simulink library "dfr"  (Simulink 8.2)
settings: Solver=ode45  SolverMode=SingleTasking  StartTime=0.0  StopTime=10.0  RelTol=1e-3
undefined symbols (not defined in the file or in its folder): ENUM_FCWSTATE_HAPTIC_ON, FALSE, KJUD_ACCMaxTimeGap_s, KJUD_ACCMediumTimeGap_s, KJUD_ACCMinTimeGap_s, KJUD_ACCShortTimeGap_s
libraries: simulink x3
settings Model: Creator=13192  LastModifiedBy=14069

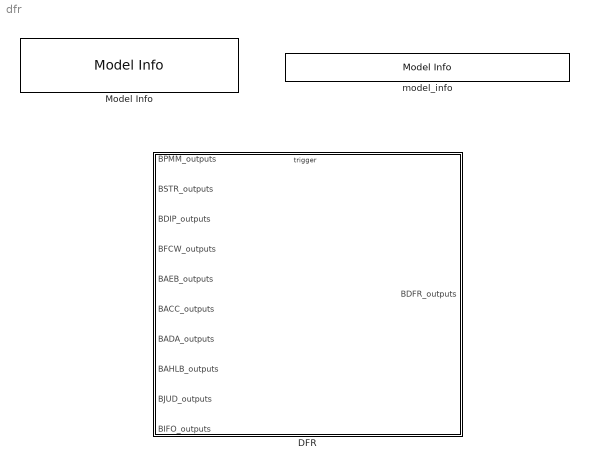
== system dfr ==
  DFR : Subsystem
      settings: RTWSystemCode=Nonreusable function  RTWFcnNameOpts=Use subsystem name  RTWFileNameOpts=Use subsystem name
  Model Info : simulink/Model-Wide Utilities/Model Info  InitialBlockCM=None  BlockCM=None  Frame=on  DisplayStringWithTags=|  HorizontalTextAlignment=Left  LeftAlignmentValue=0.02  SourceBlockDiagram=dfr  TagMaxNumber=20
      | Model Version        : %<ModelVersion>
      | Creator                   : %<Creator>
      | Last Modified by    : %<LastModifiedBy>
  model_info : simulink/Model-Wide Utilities/Model Info  InitialBlockCM=None  BlockCM=None  Frame=on  DisplayStringWithTags=$Id: hcu_lib.mdl 289 2016-04-11 06:01:08Z chimotsai $  HorizontalTextAlignment=Center  LeftAlignmentValue=0.5  SourceBlockDiagram=dfr  TagMaxNumber=20

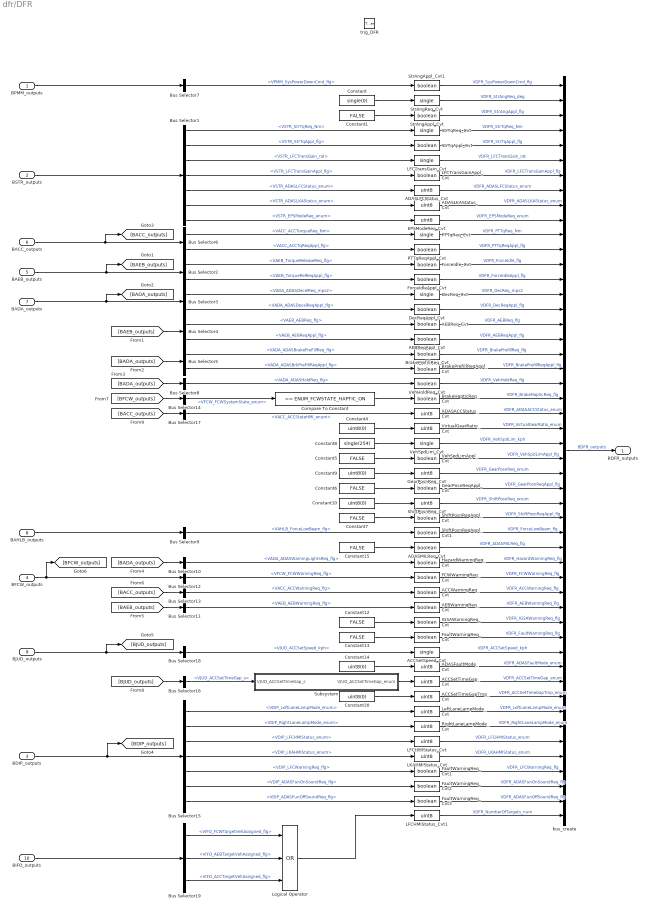
== system dfr/DFR ==
  BPMM_outputs : Inport  OutDataTypeStr=Bus: BPMM_outputs
  BSTR_outputs : Inport  Port=2  OutDataTypeStr=Bus: BSTR_outputs
  BDIP_outputs : Inport  Port=3  OutDataTypeStr=Bus: BDIP_outputs
  BFCW_outputs : Inport  Port=4  OutDataTypeStr=Bus: BFCW_outputs
  BAEB_outputs : Inport  Port=5  OutDataTypeStr=Bus: BAEB_outputs
  BACC_outputs : Inport  Port=6  OutDataTypeStr=Bus: BACC_outputs
  BADA_outputs : Inport  Port=7  OutDataTypeStr=Bus: BADA_outputs
  BAHLB_outputs : Inport  Port=8  OutDataTypeStr=Bus: BAHLB_outputs
  BJUD_outputs : Inport  Port=9  OutDataTypeStr=Bus: BJUD_outputs
  BIFO_outputs : Inport  Port=10  OutDataTypeStr=Bus: BIFO_outputs
  trig_DFR : TriggerPort  TriggerType=function-call
  ACCSetSpeed_Cvt : DataTypeConversion  OutDataTypeStr=single  SaturateOnIntegerOverflow=on  RndMeth=Zero
  ACCSetTimeGapTmp_Cvt : DataTypeConversion  OutDataTypeStr=uint8  SaturateOnIntegerOverflow=on  RndMeth=Zero
  ACCSetTimeGap_Cvt : DataTypeConversion  OutDataTypeStr=uint8  SaturateOnIntegerOverflow=on  RndMeth=Zero
  ACCWarningReq_Cvt : DataTypeConversion  OutDataTypeStr=boolean  SaturateOnIntegerOverflow=on  RndMeth=Zero
  ADASACCStatus_Cvt : DataTypeConversion  OutDataTypeStr=uint8  SaturateOnIntegerOverflow=on  RndMeth=Zero
  ADASFaultMode_Cvt : DataTypeConversion  OutDataTypeStr=uint8  SaturateOnIntegerOverflow=on  RndMeth=Zero
  ADASLFCStatus_Cvt : DataTypeConversion  OutDataTypeStr=uint8  SaturateOnIntegerOverflow=on  RndMeth=Zero
  ADASLKAStatus_Cvt : DataTypeConversion  OutDataTypeStr=uint8  SaturateOnIntegerOverflow=on  RndMeth=Zero
  ADASMILReq_Cvt : DataTypeConversion  OutDataTypeStr=boolean  SaturateOnIntegerOverflow=on  RndMeth=Zero
  AEBReqAppl_Cvt : DataTypeConversion  OutDataTypeStr=boolean  SaturateOnIntegerOverflow=on  RndMeth=Zero
  AEBReq_Cvt : DataTypeConversion  OutDataTypeStr=boolean  SaturateOnIntegerOverflow=on  RndMeth=Zero
  AEBWarningReq_Cvt : DataTypeConversion  OutDataTypeStr=boolean  SaturateOnIntegerOverflow=on  RndMeth=Zero
  BrakeHapticReq_Cvt : DataTypeConversion  OutDataTypeStr=boolean  SaturateOnIntegerOverflow=on  RndMeth=Zero
  BrakePrefillReqAppl_Cvt : DataTypeConversion  OutDataTypeStr=boolean  SaturateOnIntegerOverflow=on  RndMeth=Zero
  BrakePrefillReq_Cvt : DataTypeConversion  OutDataTypeStr=boolean  SaturateOnIntegerOverflow=on  RndMeth=Zero
  Bus Selector1 : BusSelector  OutputSignals=VSTR_StrTqReq_Nm,VSTR_StrTqAppl_flg,VSTR_LFCTransGain_rat,VSTR_LFCTransGainAppl_flg,VSTR_ADASLFCStatus_enum,VSTR_ADASLKAStatus_enum,VSTR_EPSModeReq_enum
  Bus Selector10 : BusSelector  OutputSignals=VADA_ADASWarningLightsReq_flg
  Bus Selector11 : BusSelector  OutputSignals=VAEB_AEBWarningReq_flg
  Bus Selector12 : BusSelector  OutputSignals=VFCW_FCWWarningReq_flg
  Bus Selector13 : BusSelector  OutputSignals=VACC_ACCWarningReq_flg
  Bus Selector14 : BusSelector  OutputSignals=VFCW_FCWSystemState_enum
  Bus Selector15 : BusSelector  OutputSignals=VDIP_LeftLaneLampMode_enum,VDIP_RightLaneLampMode_enum,VDIP_LFCHMIStatus_enum,VDIP_LKAHMIStatus_enum,VDIP_LFCWarningReq_flg,VDIP_ADASFunOnSoundReq_flg,VDIP_ADASFunOffSoundReq_flg
  Bus Selector16 : BusSelector  OutputSignals=VJUD_ACCSetTimeGap_s
  Bus Selector17 : BusSelector  OutputSignals=VACC_ACCStateHMI_enum
  Bus Selector18 : BusSelector  OutputSignals=VJUD_ACCSetSpeed_kph
  Bus Selector19 : BusSelector  OutputSignals=VIFO_FCWTargetVehAssigned_flg,VIFO_AEBTargetVehAssigned_flg,VIFO_ACCTargetVehAssigned_flg
  Bus Selector2 : BusSelector  OutputSignals=VAEB_TorqueReleaseReq_flg,VAEB_TorqueRelReqAppl_flg
  Bus Selector3 : BusSelector  OutputSignals=VADA_ADASDecelReq_mps2,VADA_ADASDecelReqAppl_flg
  Bus Selector4 : BusSelector  OutputSignals=VAEB_AEBReq_flg,VAEB_AEBReqAppl_flg
  Bus Selector5 : BusSelector  OutputSignals=VADA_ADASBrakePreFillReq_flg,VADA_ADASBrkPreFillReqAppl_flg
  Bus Selector6 : BusSelector  OutputSignals=VACC_ACCTorqueReq_Nm,VACC_ACCTqReqAppl_flg
  Bus Selector7 : BusSelector  OutputSignals=VPMM_SysPowerDownCmd_flg
  Bus Selector8 : BusSelector  OutputSignals=VADA_ADASHoldReq_flg
  Bus Selector9 : BusSelector  OutputSignals=VAHLB_ForceLowBeam_flg
  Compare To Constant : simulink/Logic and Bit Operations/Compare To Constant  relop===  const=ENUM_FCWSTATE_HAPTIC_ON  OutDataTypeStr=boolean
  Constant : Constant  Value=single(0)
  Constant{1,5..7,12..13,15} (7 alike) : Constant  Value=FALSE
  Constant{4,9..10,14,20} (5 alike) : Constant  Value=uint8(0)
  Constant8 : Constant  Value=single(254)
  DecReqAppl_Cvt : DataTypeConversion  OutDataTypeStr=boolean  SaturateOnIntegerOverflow=on  RndMeth=Zero
  DecReq_Cvt : DataTypeConversion  OutDataTypeStr=single  SaturateOnIntegerOverflow=on  RndMeth=Zero
  EPSModeReq_Cvt : DataTypeConversion  OutDataTypeStr=uint8  SaturateOnIntegerOverflow=on  RndMeth=Zero
  FCWWarningReq_Cvt : DataTypeConversion  OutDataTypeStr=boolean  SaturateOnIntegerOverflow=on  RndMeth=Zero
  FaultWarningReq_Cvt{,1..3} (4 alike) : DataTypeConversion  OutDataTypeStr=boolean  SaturateOnIntegerOverflow=on  RndMeth=Zero
  ForceIdleAppl_Cvt : DataTypeConversion  OutDataTypeStr=boolean  SaturateOnIntegerOverflow=on  RndMeth=Zero
  ForceIdle_Cvt : DataTypeConversion  OutDataTypeStr=boolean  SaturateOnIntegerOverflow=on  RndMeth=Zero
  GearPosnReqAppl_Cvt : DataTypeConversion  OutDataTypeStr=boolean  SaturateOnIntegerOverflow=on  RndMeth=Zero
  GearPosnReq_Cvt : DataTypeConversion  OutDataTypeStr=uint8  SaturateOnIntegerOverflow=on  RndMeth=Zero
  HazardWarningReq_Cvt : DataTypeConversion  OutDataTypeStr=boolean  SaturateOnIntegerOverflow=on  RndMeth=Zero
  IGSAWarningReq_Cvt : DataTypeConversion  OutDataTypeStr=boolean  SaturateOnIntegerOverflow=on  RndMeth=Zero
  LFCHMIStatus_Cvt : DataTypeConversion  OutDataTypeStr=uint8  SaturateOnIntegerOverflow=on  RndMeth=Zero
  LFCHMIStatus_Cvt1 : DataTypeConversion  OutDataTypeStr=uint8  SaturateOnIntegerOverflow=on  RndMeth=Zero
  LFCTransGainAppl_Cvt : DataTypeConversion  OutDataTypeStr=boolean  SaturateOnIntegerOverflow=on  RndMeth=Zero
  LFCTransGain_Cvt : DataTypeConversion  OutDataTypeStr=single  SaturateOnIntegerOverflow=on  RndMeth=Zero
  LKAHMIStatus_Cvt : DataTypeConversion  OutDataTypeStr=uint8  SaturateOnIntegerOverflow=on  RndMeth=Zero
  LeftLaneLampMode_Cvt : DataTypeConversion  OutDataTypeStr=uint8  SaturateOnIntegerOverflow=on  RndMeth=Zero
  Logical Operator : Logic  Operator=OR  Inputs=3  AllPortsSameDT=off  OutDataTypeStr=boolean
  PTTqReqAppl_Cvt : DataTypeConversion  OutDataTypeStr=boolean  SaturateOnIntegerOverflow=on  RndMeth=Zero
  PTTqReq_Cvt : DataTypeConversion  OutDataTypeStr=single  SaturateOnIntegerOverflow=on  RndMeth=Zero
  RightLaneLampMode_Cvt : DataTypeConversion  OutDataTypeStr=uint8  SaturateOnIntegerOverflow=on  RndMeth=Zero
  ShiftPosnReqAppl_Cvt : DataTypeConversion  OutDataTypeStr=boolean  SaturateOnIntegerOverflow=on  RndMeth=Zero
  ShiftPosnReqAppl_Cvt1 : DataTypeConversion  OutDataTypeStr=boolean  SaturateOnIntegerOverflow=on  RndMeth=Zero
  ShiftPosnReq_Cvt : DataTypeConversion  OutDataTypeStr=uint8  SaturateOnIntegerOverflow=on  RndMeth=Zero
  StrAngAppl_Cvt : DataTypeConversion  OutDataTypeStr=boolean  SaturateOnIntegerOverflow=on  RndMeth=Zero
  StrAngAppl_Cvt1 : DataTypeConversion  OutDataTypeStr=boolean  SaturateOnIntegerOverflow=on  RndMeth=Zero
  StrAngReq_Cvt : DataTypeConversion  OutDataTypeStr=single  SaturateOnIntegerOverflow=on  RndMeth=Zero
  StrTqAppl_Cvt : DataTypeConversion  OutDataTypeStr=boolean  SaturateOnIntegerOverflow=on  RndMeth=Zero
  StrTqReq_Cvt : DataTypeConversion  OutDataTypeStr=single  SaturateOnIntegerOverflow=on  RndMeth=Zero
  Subsystem : Subsystem
  VehHoldReq_Cvt : DataTypeConversion  OutDataTypeStr=boolean  SaturateOnIntegerOverflow=on  RndMeth=Zero
  VehSpdLimAppl_Cvt : DataTypeConversion  OutDataTypeStr=boolean  SaturateOnIntegerOverflow=on  RndMeth=Zero
  VehSpdLim_Cvt : DataTypeConversion  OutDataTypeStr=single  SaturateOnIntegerOverflow=on  RndMeth=Zero
  VirtualGearRatio_Cvt : DataTypeConversion  OutDataTypeStr=uint8  SaturateOnIntegerOverflow=on  RndMeth=Zero
  bus_create : BusCreator  Inputs=50  OutDataTypeStr=Bus: BDFR_outputs
  BDFR_outputs : Outport  OutDataTypeStr=Bus: BDFR_outputs
  wires:
  Bus Selector19/2 -> Logical Operator/2  "<VIFO_AEBTargetVehAssigned_flg>"
  Bus Selector19/1 -> Logical Operator/1  "<VIFO_FCWTargetVehAssigned_flg>"
  Bus Selector19/3 -> Logical Operator/3  "<VIFO_ACCTargetVehAssigned_flg>"
  BIFO_outputs/1 -> Bus Selector19/1
  Logical Operator/1 -> LFCHMIStatus_Cvt1/1
  Bus Selector14/1 -> Compare To Constant/1  "<VFCW_FCWSystemState_enum>"
  [BFCW_outputs] -> Bus Selector14/1
  Subsystem/1(VJUD_ACCSetTimeGap_enum) -> ACCSetTimeGap_Cvt/1
  Bus Selector18/1 -> ACCSetSpeed_Cvt/1  "<VJUD_ACCSetSpeed_kph>"
  BJUD_outputs/1 -> [BJUD_outputs], Bus Selector18/1
  [BACC_outputs] -> Bus Selector17/1
  [BJUD_outputs] -> Bus Selector16/1
  BSTR_outputs/1 -> Bus Selector1/1
  BDIP_outputs/1 -> Bus Selector15/1, [BDIP_outputs]
  BPMM_outputs/1 -> Bus Selector7/1
  bus_create/1 -> BDFR_outputs/1  "BDFR_outputs"
  StrAngReq_Cvt/1 -> bus_create/2  "VDFR_StrAngReq_deg"
  StrAngAppl_Cvt/1 -> bus_create/3  "VDFR_StrAngAppl_flg"
  StrTqReq_Cvt/1 -> bus_create/4  "VDFR_StrTqReq_Nm"
  StrTqAppl_Cvt/1 -> bus_create/5  "VDFR_StrTqAppl_flg"
  LFCTransGain_Cvt/1 -> bus_create/6  "VDFR_LFCTransGain_rat"
  LFCTransGainAppl_Cvt/1 -> bus_create/7  "VDFR_LFCTransGainAppl_flg"
  ADASLFCStatus_Cvt/1 -> bus_create/8  "VDFR_ADASLFCStatus_enum"
  ADASLKAStatus_Cvt/1 -> bus_create/9  "VDFR_ADASLKAStatus_enum"
  EPSModeReq_Cvt/1 -> bus_create/10  "VDFR_EPSModeReq_enum"
  PTTqReq_Cvt/1 -> bus_create/11  "VDFR_PTTqReq_Nm"
  ForceIdle_Cvt/1 -> bus_create/13  "VDFR_ForceIdle_flg"
  PTTqReqAppl_Cvt/1 -> bus_create/12  "VDFR_PTTqReqAppl_flg"
  DecReqAppl_Cvt/1 -> bus_create/16  "VDFR_DecReqAppl_flg"
  ForceIdleAppl_Cvt/1 -> bus_create/14  "VDFR_ForceIdleAppl_flg"
  DecReq_Cvt/1 -> bus_create/15  "VDFR_DecReq_mps2"
  AEBReq_Cvt/1 -> bus_create/17  "VDFR_AEBReq_flg"
  AEBReqAppl_Cvt/1 -> bus_create/18  "VDFR_AEBReqAppl_flg"
  BrakePrefillReq_Cvt/1 -> bus_create/19  "VDFR_BrakePrefillReq_flg"
  BrakePrefillReqAppl_Cvt/1 -> bus_create/20  "VDFR_BrakePrefillReqAppl_flg"
  VehHoldReq_Cvt/1 -> bus_create/21  "VDFR_VehHoldReq_flg"
  BrakeHapticReq_Cvt/1 -> bus_create/22  "VDFR_BrakeHapticReq_flg"
  ADASACCStatus_Cvt/1 -> bus_create/23  "VDFR_ADASACCStatus_enum"
  VirtualGearRatio_Cvt/1 -> bus_create/24  "VDFR_VirtualGearRatio_enum"
  VehSpdLim_Cvt/1 -> bus_create/25  "VDFR_VehSpdLim_kph"
  VehSpdLimAppl_Cvt/1 -> bus_create/26  "VDFR_VehSpdLimAppl_flg"
  GearPosnReq_Cvt/1 -> bus_create/27  "VDFR_GearPosnReq_enum"
  GearPosnReqAppl_Cvt/1 -> bus_create/28  "VDFR_GearPosnReqAppl_flg"
  ShiftPosnReq_Cvt/1 -> bus_create/29  "VDFR_ShiftPosnReq_enum"
  ShiftPosnReqAppl_Cvt/1 -> bus_create/30  "VDFR_ShiftPosnReqAppl_flg"
  ADASMILReq_Cvt/1 -> bus_create/32  "VDFR_ADASMILReq_flg"
  HazardWarningReq_Cvt/1 -> bus_create/33  "VDFR_HazardWarningReq_flg"
  FCWWarningReq_Cvt/1 -> bus_create/34  "VDFR_FCWWarningReq_flg"
  ACCWarningReq_Cvt/1 -> bus_create/35  "VDFR_ACCWarningReq_flg"
  AEBWarningReq_Cvt/1 -> bus_create/36  "VDFR_AEBWarningReq_flg"
  IGSAWarningReq_Cvt/1 -> bus_create/37  "VDFR_IGSAWarningReq_flg"
  FaultWarningReq_Cvt/1 -> bus_create/38  "VDFR_FaultWarningReq_flg"
  ACCSetSpeed_Cvt/1 -> bus_create/39  "VDFR_ACCSetSpeed_kph"
  ADASFaultMode_Cvt/1 -> bus_create/40  "VDFR_ADASFaultMode_enum"
  ACCSetTimeGap_Cvt/1 -> bus_create/41  "VDFR_ACCSetTimeGap_enum"
  ACCSetTimeGapTmp_Cvt/1 -> bus_create/42  "VDFR_ACCSetTimeGapTmp_enum"
  LeftLaneLampMode_Cvt/1 -> bus_create/43  "VDFR_LeftLaneLampMode_enum"
  RightLaneLampMode_Cvt/1 -> bus_create/44  "VDFR_RightLaneLampMode_enum"
  LFCHMIStatus_Cvt/1 -> bus_create/45  "VDFR_LFCHMIStatus_enum"
  LKAHMIStatus_Cvt/1 -> bus_create/46  "VDFR_LKAHMIStatus_enum"
  Bus Selector1/4 -> LFCTransGainAppl_Cvt/1  "<VSTR_LFCTransGainAppl_flg>"
  Bus Selector1/5 -> ADASLFCStatus_Cvt/1  "<VSTR_ADASLFCStatus_enum>"
  Bus Selector1/3 -> LFCTransGain_Cvt/1  "<VSTR_LFCTransGain_rat>"
  Bus Selector1/6 -> ADASLKAStatus_Cvt/1  "<VSTR_ADASLKAStatus_enum>"
  Bus Selector1/2 -> StrTqAppl_Cvt/1  "<VSTR_StrTqAppl_flg>"
  Bus Selector1/1 -> StrTqReq_Cvt/1  "<VSTR_StrTqReq_Nm>"
  Bus Selector1/7 -> EPSModeReq_Cvt/1  "<VSTR_EPSModeReq_enum>"
  Constant/1 -> StrAngReq_Cvt/1
  Constant1/1 -> StrAngAppl_Cvt/1
  Bus Selector7/1 -> StrAngAppl_Cvt1/1  "<VPMM_SysPowerDownCmd_flg>"
  StrAngAppl_Cvt1/1 -> bus_create/1  "VDFR_SysPowerDownCmd_flg"
  BAEB_outputs/1 -> [BAEB_outputs], Bus Selector2/1
  [BAEB_outputs] -> Bus Selector4/1
  [BADA_outputs] -> Bus Selector5/1
  [BADA_outputs] -> Bus Selector8/1
  Compare To Constant/1 -> BrakeHapticReq_Cvt/1
  Bus Selector17/1 -> ADASACCStatus_Cvt/1  "<VACC_ACCStateHMI_enum>"
  Constant4/1 -> VirtualGearRatio_Cvt/1
  Constant5/1 -> VehSpdLimAppl_Cvt/1
  Constant6/1 -> GearPosnReqAppl_Cvt/1
  Constant7/1 -> ShiftPosnReqAppl_Cvt/1
  Constant8/1 -> VehSpdLim_Cvt/1
  Constant9/1 -> GearPosnReq_Cvt/1
  Constant10/1 -> ShiftPosnReq_Cvt/1
  ShiftPosnReqAppl_Cvt1/1 -> bus_create/31  "VDFR_ForceLowBeam_flg"
  BAHLB_outputs/1 -> Bus Selector9/1
  Bus Selector9/1 -> ShiftPosnReqAppl_Cvt1/1  "<VAHLB_ForceLowBeam_flg>"
  [BADA_outputs] -> Bus Selector10/1
  [BAEB_outputs] -> Bus Selector11/1
  BFCW_outputs/1 -> Bus Selector12/1, [BFCW_outputs]
  Constant12/1 -> IGSAWarningReq_Cvt/1
  Constant13/1 -> FaultWarningReq_Cvt/1
  Constant14/1 -> ADASFaultMode_Cvt/1
  Bus Selector15/1 -> LeftLaneLampMode_Cvt/1  "<VDIP_LeftLaneLampMode_enum>"
  Bus Selector15/2 -> RightLaneLampMode_Cvt/1  "<VDIP_RightLaneLampMode_enum>"
  Bus Selector15/3 -> LFCHMIStatus_Cvt/1  "<VDIP_LFCHMIStatus_enum>"
  Bus Selector15/4 -> LKAHMIStatus_Cvt/1  "<VDIP_LKAHMIStatus_enum>"
  Constant15/1 -> ADASMILReq_Cvt/1
  FaultWarningReq_Cvt1/1 -> bus_create/47  "VDFR_LFCWarningReq_flg"
  Bus Selector15/5 -> FaultWarningReq_Cvt1/1  "<VDIP_LFCWarningReq_flg>"
  FaultWarningReq_Cvt2/1 -> bus_create/48  "VDFR_ADASFunOnSoundReq_flg"
  Bus Selector15/6 -> FaultWarningReq_Cvt2/1  "<VDIP_ADASFunOnSoundReq_flg>"
  FaultWarningReq_Cvt3/1 -> bus_create/49  "VDFR_ADASFunOffSoundReq_flg"
  Bus Selector15/7 -> FaultWarningReq_Cvt3/1  "<VDIP_ADASFunOffSoundReq_flg>"
  LFCHMIStatus_Cvt1/1 -> bus_create/50  "VDFR_NumberOfTargets_num"
  Bus Selector6/1 -> PTTqReq_Cvt/1  "<VACC_ACCTorqueReq_Nm>"
  Bus Selector2/1 -> ForceIdle_Cvt/1  "<VAEB_TorqueReleaseReq_flg>"
  Bus Selector2/2 -> ForceIdleAppl_Cvt/1  "<VAEB_TorqueRelReqAppl_flg>"
  Bus Selector6/2 -> PTTqReqAppl_Cvt/1  "<VACC_ACCTqReqAppl_flg>"
  BADA_outputs/1 -> [BADA_outputs], Bus Selector3/1
  Bus Selector3/1 -> DecReq_Cvt/1  "<VADA_ADASDecelReq_mps2>"
  Bus Selector3/2 -> DecReqAppl_Cvt/1  "<VADA_ADASDecelReqAppl_flg>"
  Bus Selector4/1 -> AEBReq_Cvt/1  "<VAEB_AEBReq_flg>"
  Bus Selector4/2 -> AEBReqAppl_Cvt/1  "<VAEB_AEBReqAppl_flg>"
  Bus Selector5/1 -> BrakePrefillReq_Cvt/1  "<VADA_ADASBrakePreFillReq_flg>"
  Bus Selector5/2 -> BrakePrefillReqAppl_Cvt/1  "<VADA_ADASBrkPreFillReqAppl_flg>"
  Bus Selector8/1 -> VehHoldReq_Cvt/1  "<VADA_ADASHoldReq_flg>"
  Bus Selector10/1 -> HazardWarningReq_Cvt/1  "<VADA_ADASWarningLightsReq_flg>"
  Bus Selector12/1 -> FCWWarningReq_Cvt/1  "<VFCW_FCWWarningReq_flg>"
  Bus Selector11/1 -> AEBWarningReq_Cvt/1  "<VAEB_AEBWarningReq_flg>"
  Bus Selector16/1 -> Subsystem/1(VJUD_ACCSetTimeGap_s)  "<VJUD_ACCSetTimeGap_s>"
  Constant20/1 -> ACCSetTimeGapTmp_Cvt/1
  BACC_outputs/1 -> [BACC_outputs], Bus Selector6/1
  [BACC_outputs] -> Bus Selector13/1
  Bus Selector13/1 -> ACCWarningReq_Cvt/1  "<VACC_ACCWarningReq_flg>"

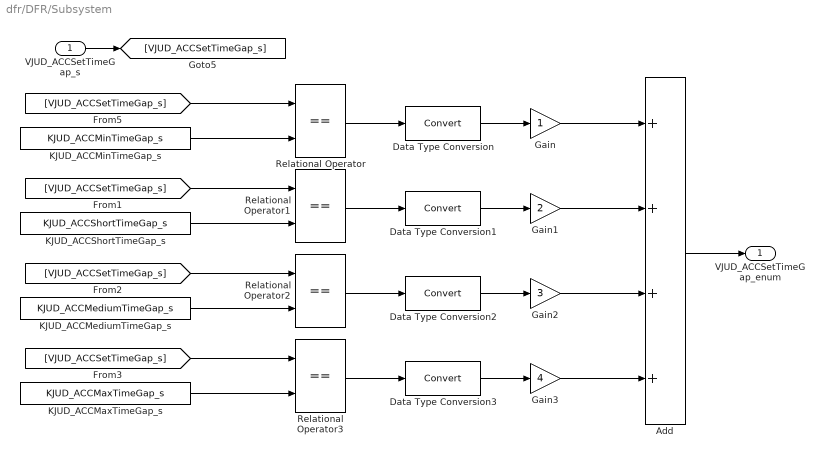
== system dfr/DFR/Subsystem ==
  VJUD_ACCSetTimeGap_s : Inport
  Add : Sum  Inputs=4
  Data Type Conversion{,1..3} (4 alike) : DataTypeConversion
  Gain : Gain
  Gain1 : Gain  Gain=2
  Gain2 : Gain  Gain=3
  Gain3 : Gain  Gain=4
  KJUD_ACCMaxTimeGap_s : Constant  Value=KJUD_ACCMaxTimeGap_s
  KJUD_ACCMediumTimeGap_s : Constant  Value=KJUD_ACCMediumTimeGap_s
  KJUD_ACCMinTimeGap_s : Constant  Value=KJUD_ACCMinTimeGap_s
  KJUD_ACCShortTimeGap_s : Constant  Value=KJUD_ACCShortTimeGap_s
  Relational Operator{,1..3} (4 alike) : RelationalOperator  Operator===  OutDataTypeStr=boolean
  VJUD_ACCSetTimeGap_enum : Outport
  wires:
  Add/1 -> VJUD_ACCSetTimeGap_enum/1
  Data Type Conversion3/1 -> Gain3/1
  Gain3/1 -> Add/4
  Relational Operator3/1 -> Data Type Conversion3/1
  [VJUD_ACCSetTimeGap_s] -> Relational Operator3/1
  KJUD_ACCMaxTimeGap_s/1 -> Relational Operator3/2
  Data Type Conversion2/1 -> Gain2/1
  Gain2/1 -> Add/3
  Relational Operator2/1 -> Data Type Conversion2/1
  [VJUD_ACCSetTimeGap_s] -> Relational Operator2/1
  KJUD_ACCMediumTimeGap_s/1 -> Relational Operator2/2
  Data Type Conversion1/1 -> Gain1/1
  Gain1/1 -> Add/2
  Relational Operator1/1 -> Data Type Conversion1/1
  [VJUD_ACCSetTimeGap_s] -> Relational Operator1/1
  KJUD_ACCShortTimeGap_s/1 -> Relational Operator1/2
  Data Type Conversion/1 -> Gain/1
  Gain/1 -> Add/1
  Relational Operator/1 -> Data Type Conversion/1
  [VJUD_ACCSetTimeGap_s] -> Relational Operator/1
  KJUD_ACCMinTimeGap_s/1 -> Relational Operator/2
  VJUD_ACCSetTimeGap_s/1 -> [VJUD_ACCSetTimeGap_s]
